simulink model "PID_Yaw_2018b"  (R2023a)
settings: Solver=ode3  StartTime=0.0  StopTime=inf  FixedStep=.02  RelTol=1e-3  EnableMultiTasking=on
InitFcn:
  | close all
  | clear
  | clc
  | Parameter_Modeling
  | ST=0.02;
  | angle_scale=.0109863;  % 1/91.0222
  | time_scale=.01;
values from neighbouring files (symbols this model uses):
  b = 1.10794e-05    [disturbance result.mat]
  d = reshape([p1dot;p2dot],2 * n^2,1)    [OpenLoop_LQDG_riccati_solver_pitch.m]    (also in OpenLoop_LQDG_riccati_solver_roll.m; disturbance result.mat = 3.2e-06)
undefined symbols (not defined in the file or in its folder): dcg, I_XX, I_YY, I_ZZ, rad, s
libraries: arduinolib x5, aerolibconvert2 x5
settings Model: SimulationMode=external  ExtModeTrigDuration=2  Creator=Alireza  LastModifiedBy=Ali
settings SolverCC: AlgebraicLoopSolver=TrustRegion
settings DataIOCC: LimitDataPoints=on  SaveFormat=Array  ReturnWorkspaceOutputs=off
settings OptimizationCC: ExpressionDepthLimit=2147483647  MaxStackSize=64  EfficientTunableParamExpr=on
settings DebuggingCC: UnderspecifiedInitializationDetection=Classic  MergeDetectMultiDrivingBlocksExec=none  ParameterTunabilityLossMsg=error  UnconnectedInputMsg=warning  UnconnectedOutputMsg=warning  UnconnectedLineMsg=warning  StateNameClashWarn=warning  SFUnexpectedBacktrackingDiag=warning  SFNoUnconditionalDefaultTransitionDiag=warning  SFExecutionAtInitializationDiag=none  ArithmeticOperatorsInVariantConditions=warning
settings HardwareCC: ProdBitPerInt=16  ProdBitPerPointer=16  ProdBitPerSizeT=16  ProdBitPerPtrDiffT=16  ProdLargestAtomicFloat=None  ProdWordSize=8  ProdHWDeviceType=Atmel->AVR
settings ModelReferenceCC: EnableRefExpFcnMdlSchedulingChecks=on  PropagateSignalLabelsOutOfModel=off
settings SFSimCC: SimUseLocalCustomCode=off  MATLABDynamicMemAlloc=off  CustomCodeUndefinedFunction=UseInterfaceOnly
settings RTWCC: Description=Embedded Coder  SystemTargetFile=ert.tlc  HardwareBoard=Arduino Mega 2560  TLCOptions=-aInlineSetEventsForThisBaseRateFcn=TLC_FALSE -aRateBasedStepFcn=1 -aSuppressMultiTaskScheduler=TLC_FALSE  TemplateMakefile=ert_default_tmf  GenerateReport=on  RTWVerbose=off  RTWUseLocalCustomCode=off  Toolchain=Arduino AVR  BuildConfiguration=Faster Runs  IncludeHyperlinkInReport=on  LaunchReport=on  GenerateTraceInfo=on  GenerateTraceReport=on  GenerateTraceReportSl=on  GenerateTraceReportSf=on  GenerateTraceReportEml=on
settings CodeAppCC: ForceParamTrailComments=on  IgnoreCustomStorageClasses=off  OperatorAnnotations=on  SimulinkDataObjDesc=on  SFDataObjDesc=on  MATLABFcnDesc=on  CustomSymbolStrType=$N$R$M  InsertBlockDesc=on  StateflowObjectComments=on  MATLABSourceComments=on  InternalIdentifier=Classic
settings ERTTargetCC: MultiwordLength=2048  SupportContinuousTime=on  SupportVariableSizeSignals=on
settings ConfigComp: CovMetricSettings=dw  CovSaveCumulativeToWorkspaceVar=on  CovSaveSingleToWorkspaceVar=on  CovExternalEMLEnable=off  CovSFcnEnable=off

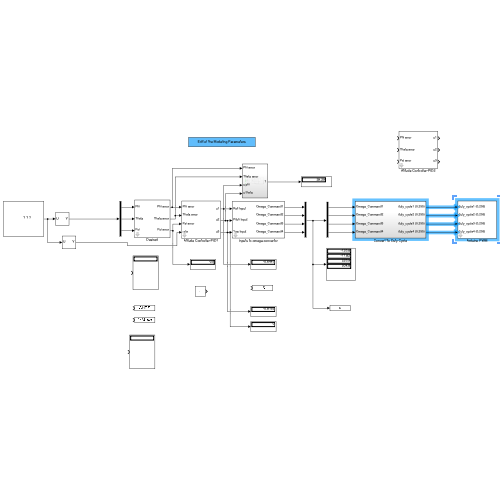
[thumbnail: Simulink's stored preview of the top-level diagram]
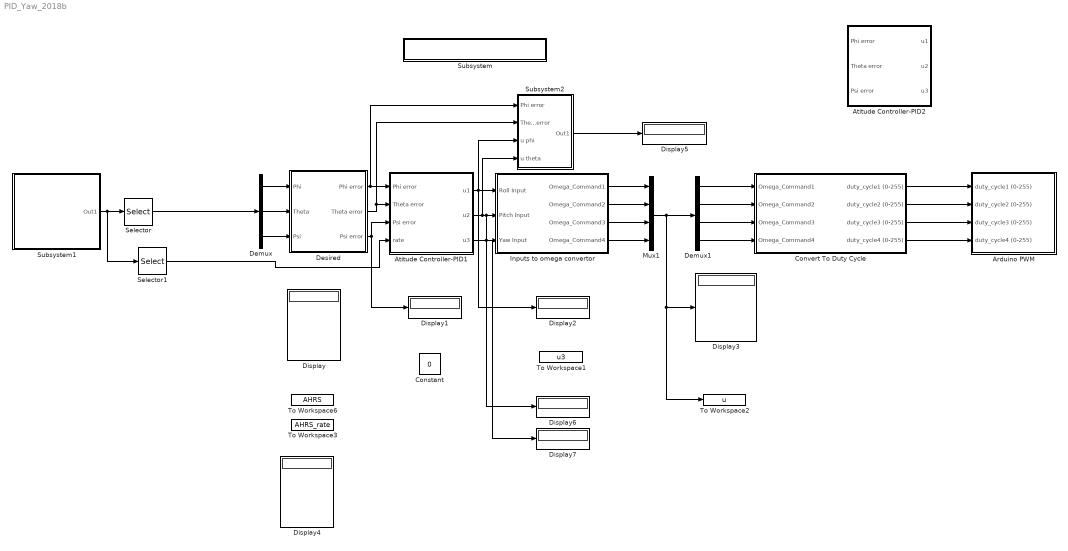
== system PID_Yaw_2018b ==
  Arduino PWM : Subsystem  mask{Motor1=8, Motor2=9, Motor3=10, Motor4=11}
      mask prompts: Motor1 "Motor 1 Pin Number"; Motor2 "Motor 2 Pin Number"; Motor3 "Motor 3 Pin Number"; Motor4 "Motor 4 Pin Number"
  Atitude Controller-PID1 : Subsystem  mask{KP_Roll=0.7, KI_Roll=0.5, KD_Roll=0.4, KP_Pitch=0.8, KI_Pitch=0.6, KD_Pitch=0.5, KP_Yaw=0, KI_Yaw=0, KD_Yaw=0}
      mask DialogControl tab1 Prompt: Roll
      mask DialogControl tab2 Prompt: Pitch
      mask DialogControl tab3 Prompt: Yaw
  Atitude Controller-PID2 : Subsystem  mask{KP_Roll=0.7, KI_Roll=0.5, KD_Roll=.4, KP_Pitch=.8, KI_Pitch=0.5, KD_Pitch=.4, KP_Yaw=0, KI_Yaw=0, KD_Yaw=0}
      mask DialogControl tab1 Prompt: Roll
      mask DialogControl tab2 Prompt: Pitch
      mask DialogControl tab3 Prompt: Yaw
  Constant : Constant  Value=0
  Convert To Duty Cycle : Subsystem
  Demux : Demux  Outputs=3
  Demux1 : Demux
  Desired : Subsystem  mask{Phi_Des=0, Theta_Des=0, Psi_Des=0}
      mask prompts: Phi_Des "Desired Phi (Degree)"; Theta_Des "Desired Theta (Degree)"; Psi_Des "Desired Psi (Degree)"
  Display{,1..7} (8 alike) : Display
  Inputs to omega convertor : Subsystem  mask{mean_rpm=2000}
  Mux1 : Mux
  Selector : Selector  InputPortWidth=6  IndexOptions=Index vector (dialog)  Indices=[1 2 3]  OutputSizes=1
  Selector1 : Selector  InputPortWidth=6  IndexOptions=Index vector (dialog)  Indices=[4 5 6]  OutputSizes=1
  Subsystem : Subsystem
      settings: OpenFcn=open('Parameter_Modeling')
      mask Display: disp('Edit of the Modeling Parameters')
  Subsystem1 : Subsystem
      mask Display: image('UM7.jpg'); % Use "Edit Image" on toolstrip to change.
  Subsystem2 : Subsystem
  To Workspace1 : ToWorkspace  VariableName=u3  SampleTime=-1
  To Workspace2 : ToWorkspace  VariableName=u  SampleTime=-1
  To Workspace3 : ToWorkspace  VariableName=AHRS_rate  SampleTime=-1
  To Workspace6 : ToWorkspace  VariableName=AHRS  SampleTime=-1
  wires:
  Desired/1(Phi error) -> Subsystem2/1(Phi error), Atitude Controller-PID1/1(Phi error)
  Desired/2(Theta error) -> Subsystem2/2(Theta error), Atitude Controller-PID1/2(Theta error)
  Desired/3(Psi error) -> Display1/1, Atitude Controller-PID1/3(Psi error)
  Convert To Duty Cycle/3(duty_cycle3 (0-255)) -> Arduino PWM/3(duty_cycle3 (0-255))
  Convert To Duty Cycle/1(duty_cycle1 (0-255)) -> Arduino PWM/1(duty_cycle1 (0-255))
  Convert To Duty Cycle/4(duty_cycle4 (0-255)) -> Arduino PWM/4(duty_cycle4 (0-255))
  Convert To Duty Cycle/2(duty_cycle2 (0-255)) -> Arduino PWM/2(duty_cycle2 (0-255))
  Demux/2 -> Desired/2(Theta)
  Demux/1 -> Desired/1(Phi)
  Demux/3 -> Desired/3(Psi)
  Mux1/1 -> Demux1/1, To Workspace2/1, Display3/1
  Inputs to omega convertor/2(Omega_Command2) -> Mux1/2
  Inputs to omega convertor/4(Omega_Command4) -> Mux1/4
  Inputs to omega convertor/3(Omega_Command3) -> Mux1/3
  Inputs to omega convertor/1(Omega_Command1) -> Mux1/1
  Demux1/4 -> Convert To Duty Cycle/4(Omega_Command4)
  Demux1/2 -> Convert To Duty Cycle/2(Omega_Command2)
  Demux1/3 -> Convert To Duty Cycle/3(Omega_Command3)
  Demux1/1 -> Convert To Duty Cycle/1(Omega_Command1)
  Subsystem1/1(Out1) -> Selector1/1, Selector/1
  Selector1/1 -> Atitude Controller-PID1/4(rate)
  Atitude Controller-PID1/1(u1) -> Display2/1, Subsystem2/3(u phi), Inputs to omega convertor/1(Roll Input)
  Atitude Controller-PID1/2(u2) -> Subsystem2/4(u theta), Display6/1, Inputs to omega convertor/2(Pitch Input)
  Atitude Controller-PID1/3(u3) -> Display7/1, Inputs to omega convertor/3(Yaw Input)
  Subsystem2/1(Out1) -> Display5/1
  Selector/1 -> Demux/1

== system PID_Yaw_2018b/Arduino PWM ==
  duty_cycle1 (0-255) : Inport
  duty_cycle2 (0-255) : Inport  Port=2
  duty_cycle3 (0-255) : Inport  Port=3
  duty_cycle4 (0-255) : Inport  Port=4
  PWM : arduinolib/PWM  pinNumber=8  frequencyType=Default  desiredFrequency=490.2  achievableFrequency=490.2
  PWM1 : arduinolib/PWM  pinNumber=9  frequencyType=Default  desiredFrequency=490.2  achievableFrequency=490.2
  PWM2 : arduinolib/PWM  pinNumber=10  frequencyType=Default  desiredFrequency=490.2  achievableFrequency=490.2
  PWM3 : arduinolib/PWM  pinNumber=11  frequencyType=Default  desiredFrequency=490.2  achievableFrequency=490.2
  wires:
  duty_cycle1 (0-255)/1 -> PWM/1
  duty_cycle2 (0-255)/1 -> PWM1/1
  duty_cycle3 (0-255)/1 -> PWM2/1
  duty_cycle4 (0-255)/1 -> PWM3/1

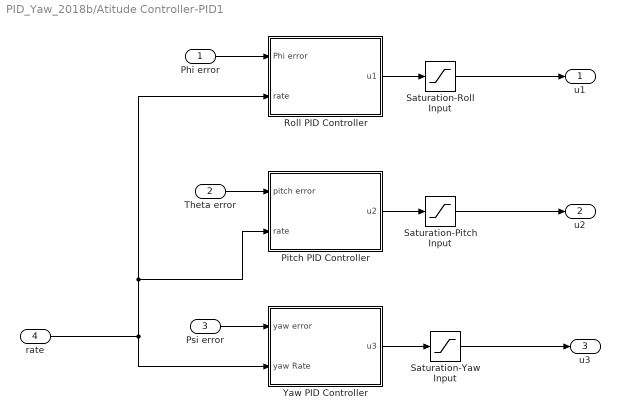
== system PID_Yaw_2018b/Atitude Controller-PID1 ==
  Phi error : Inport
  Theta error : Inport  Port=2
  Psi error : Inport  Port=3
  rate : Inport  Port=4
  Pitch PID Controller : Subsystem
  Roll PID Controller : Subsystem
  Saturation-Pitch Input : Saturate  UpperLimit=2  LowerLimit=-2
  Saturation-Roll Input : Saturate  UpperLimit=2  LowerLimit=-2
  Saturation-Yaw Input : Saturate  UpperLimit=2  LowerLimit=-2
  Yaw PID Controller : Subsystem
  u1 : Outport
  u2 : Outport  Port=2
  u3 : Outport  Port=3
  wires:
  Yaw PID Controller/1(u3) -> Saturation-Yaw Input/1
  Pitch PID Controller/1(u2) -> Saturation-Pitch Input/1
  Roll PID Controller/1(u1) -> Saturation-Roll Input/1
  Saturation-Roll Input/1 -> u1/1
  Psi error/1 -> Yaw PID Controller/1(yaw error)
  Theta error/1 -> Pitch PID Controller/1(pitch error)
  Phi error/1 -> Roll PID Controller/1(Phi error)
  rate/1 -> Pitch PID Controller/2(rate), Roll PID Controller/2(rate), Yaw PID Controller/2(yaw Rate)
  Saturation-Pitch Input/1 -> u2/1
  Saturation-Yaw Input/1 -> u3/1

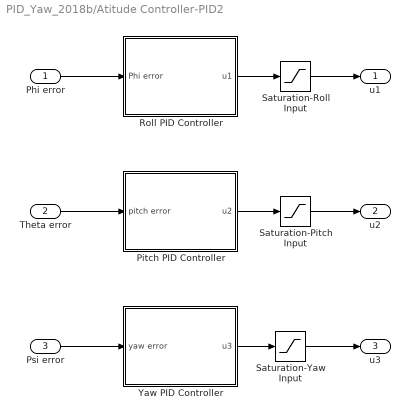
== system PID_Yaw_2018b/Atitude Controller-PID2 ==
  Phi error : Inport
  Theta error : Inport  Port=2
  Psi error : Inport  Port=3
  Pitch PID Controller : Subsystem
  Roll PID Controller : Subsystem
  Saturation-Pitch Input : Saturate  UpperLimit=2  LowerLimit=-2
  Saturation-Roll Input : Saturate  UpperLimit=2  LowerLimit=-2
  Saturation-Yaw Input : Saturate  UpperLimit=2  LowerLimit=-2
  Yaw PID Controller : Subsystem
  u1 : Outport
  u2 : Outport  Port=2
  u3 : Outport  Port=3
  wires:
  Yaw PID Controller/1(u3) -> Saturation-Yaw Input/1
  Pitch PID Controller/1(u2) -> Saturation-Pitch Input/1
  Roll PID Controller/1(u1) -> Saturation-Roll Input/1
  Saturation-Yaw Input/1 -> u3/1
  Saturation-Roll Input/1 -> u1/1
  Saturation-Pitch Input/1 -> u2/1
  Psi error/1 -> Yaw PID Controller/1(yaw error)
  Theta error/1 -> Pitch PID Controller/1(pitch error)
  Phi error/1 -> Roll PID Controller/1(Phi error)

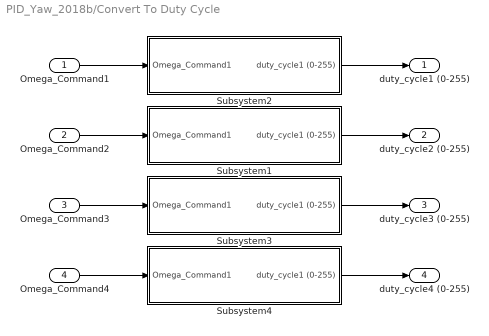
== system PID_Yaw_2018b/Convert To Duty Cycle ==
  Omega_Command1 : Inport
  Omega_Command2 : Inport  Port=2
  Omega_Command3 : Inport  Port=3
  Omega_Command4 : Inport  Port=4
  Subsystem1 : Subsystem
  Subsystem2 : Subsystem
  Subsystem3 : Subsystem
  Subsystem4 : Subsystem
  duty_cycle1 (0-255) : Outport
  duty_cycle2 (0-255) : Outport  Port=2
  duty_cycle3 (0-255) : Outport  Port=3
  duty_cycle4 (0-255) : Outport  Port=4
  wires:
  Subsystem1/1(duty_cycle1 (0-255)) -> duty_cycle2 (0-255)/1
  Subsystem3/1(duty_cycle1 (0-255)) -> duty_cycle3 (0-255)/1
  Subsystem4/1(duty_cycle1 (0-255)) -> duty_cycle4 (0-255)/1
  Subsystem2/1(duty_cycle1 (0-255)) -> duty_cycle1 (0-255)/1
  Omega_Command1/1 -> Subsystem2/1(Omega_Command1)
  Omega_Command4/1 -> Subsystem4/1(Omega_Command1)
  Omega_Command3/1 -> Subsystem3/1(Omega_Command1)
  Omega_Command2/1 -> Subsystem1/1(Omega_Command1)

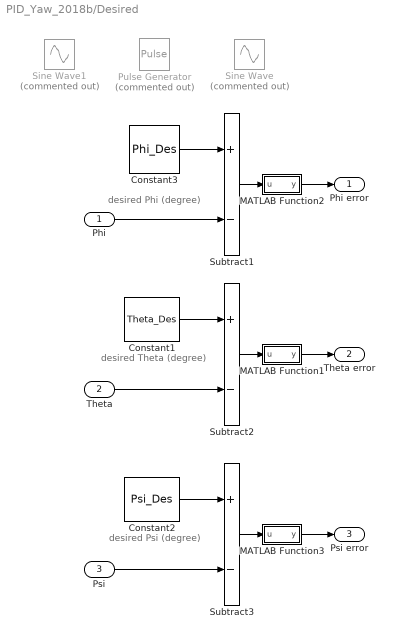
== system PID_Yaw_2018b/Desired ==
  note: desired Phi (degree)
  note: desired Theta (degree)
  note: desired Psi (degree)
  Phi : Inport
  Theta : Inport  Port=2
  Psi : Inport  Port=3
  Constant1 : Constant  Value=Theta_Des
  Constant2 : Constant  Value=Psi_Des
  Constant3 : Constant  Value=Phi_Des
  MATLAB Function1 : MATLAB Function  TreatAsAtomicUnit=on
  MATLAB Function2 : MATLAB Function  TreatAsAtomicUnit=on
  MATLAB Function3 : MATLAB Function  TreatAsAtomicUnit=on
  Pulse Generator : DiscretePulseGenerator  Commented=on  PulseType=Time based  Amplitude=20  Period=10  PulseWidth=5
  Sine Wave : Sin  Commented=on  Amplitude=10  SampleTime=0
  Sine Wave1 : Sin  Commented=on  Amplitude=20  Phase=pi/2  SampleTime=0
  Subtract1 : Sum  Inputs=+-
  Subtract2 : Sum  Inputs=+-
  Subtract3 : Sum  Inputs=+-
  Phi error : Outport
  Theta error : Outport  Port=2
  Psi error : Outport  Port=3
  wires:
  Constant2/1 -> Subtract3/1
  Psi/1 -> Subtract3/2
  Subtract2/1 -> MATLAB Function1/1(u)
  Theta/1 -> Subtract2/2
  Subtract1/1 -> MATLAB Function2/1(u)
  Phi/1 -> Subtract1/2
  Subtract3/1 -> MATLAB Function3/1(u)
  MATLAB Function2/1(y) -> Phi error/1
  MATLAB Function1/1(y) -> Theta error/1
  MATLAB Function3/1(y) -> Psi error/1
  Constant1/1 -> Subtract2/1
  Constant3/1 -> Subtract1/1

== system PID_Yaw_2018b/Inputs to omega convertor ==
  Roll Input : Inport
  Pitch Input : Inport  Port=2
  Yaw Input : Inport  Port=3
  " 1" : Constant  Value=mean_rpm
  Inputs to omega convertor : Subsystem
  Omega_Command1 : Outport
  Omega_Command2 : Outport  Port=2
  Omega_Command3 : Outport  Port=3
  Omega_Command4 : Outport  Port=4
  wires:
  " 1"/1 -> Inputs to omega convertor/1(mean rpm)
  Roll Input/1 -> Inputs to omega convertor/2(Roll Input (Roll Moment))
  Pitch Input/1 -> Inputs to omega convertor/3(Pitch Input (Pitch Moment))
  Yaw Input/1 -> Inputs to omega convertor/4(Yaw Input(Yaw Moment))
  Inputs to omega convertor/4(Omega_Command4) -> Omega_Command4/1
  Inputs to omega convertor/1(Omega_Command1) -> Omega_Command1/1
  Inputs to omega convertor/2(Omega_Command2) -> Omega_Command2/1
  Inputs to omega convertor/3(Omega_Command3) -> Omega_Command3/1

== system PID_Yaw_2018b/Subsystem ==

== system PID_Yaw_2018b/Subsystem1 ==
  AHRS : Subsystem
  Mux : Mux  Inputs=6
  Out1 : Outport
  wires:
  AHRS/2(theta) -> Mux/2
  AHRS/1(phi) -> Mux/1
  AHRS/3(psi) -> Mux/3
  AHRS/4(roll_rate) -> Mux/4
  AHRS/5(pitch_rate) -> Mux/5
  AHRS/6(yaw_rate) -> Mux/6
  Mux/1 -> Out1/1

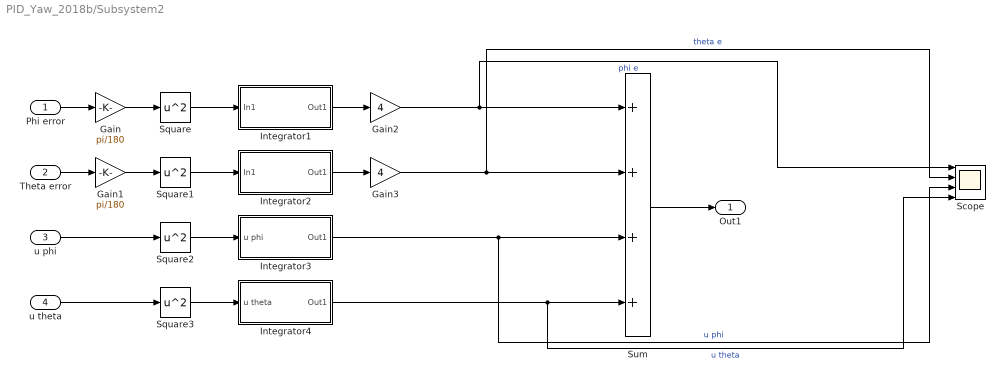
== system PID_Yaw_2018b/Subsystem2 ==
  Phi error : Inport
  Theta error : Inport  Port=2
  u phi : Inport  Port=3
  u theta : Inport  Port=4
  Gain : Gain  Gain=pi/180
  Gain1 : Gain  Gain=pi/180
  Gain2 : Gain  Gain=4
  Gain3 : Gain  Gain=4
  Integrator1 : Subsystem
  Integrator2 : Subsystem
  Integrator3 : Subsystem
  Integrator4 : Subsystem
  Scope : Scope  NumInputPorts=4
  Square{,1..3} (4 alike) : Math  Operator=square
  Sum : Sum  Inputs=++++
  Out1 : Outport
  wires:
  Sum/1 -> Out1/1
  Integrator1/1(Out1) -> Gain2/1
  Integrator2/1(Out1) -> Gain3/1
  Integrator3/1(Out1) -> Scope/3, Sum/3  "u phi"
  Integrator4/1(Out1) -> Scope/4, Sum/4  "u theta"
  Gain/1 -> Square/1
  Phi error/1 -> Gain/1
  Theta error/1 -> Gain1/1
  Gain1/1 -> Square1/1
  u phi/1 -> Square2/1
  u theta/1 -> Square3/1
  Square/1 -> Integrator1/1(In1)
  Square1/1 -> Integrator2/1(In1)
  Square2/1 -> Integrator3/1(u phi)
  Square3/1 -> Integrator4/1(u theta)
  Gain2/1 -> Scope/1, Sum/1  "phi e"
  Gain3/1 -> Scope/2, Sum/2  "theta e"

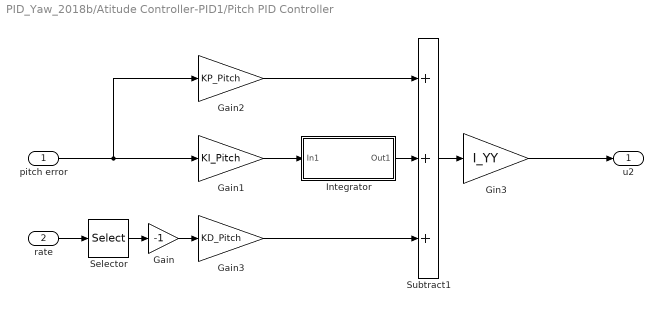
== system PID_Yaw_2018b/Atitude Controller-PID1/Pitch PID Controller ==
  pitch error : Inport
  rate : Inport  Port=2
  Gain : Gain  Gain=-1
  Gain1 : Gain  Gain=KI_Pitch
  Gain2 : Gain  Gain=KP_Pitch
  Gain3 : Gain  Gain=KD_Pitch
  Gin3 : Gain  Gain=I_YY
  Integrator : Subsystem
  Selector : Selector  InputPortWidth=3  IndexOptions=Index vector (dialog)  Indices=[2]  OutputSizes=1
  Subtract1 : Sum  Inputs=+++
  u2 : Outport
  wires:
  Integrator/1(Out1) -> Subtract1/2
  Gain1/1 -> Integrator/1(In1)
  Gain2/1 -> Subtract1/1
  Subtract1/1 -> Gin3/1
  Gain/1 -> Gain3/1
  pitch error/1 -> Gain1/1, Gain2/1
  Gin3/1 -> u2/1
  Gain3/1 -> Subtract1/3
  rate/1 -> Selector/1
  Selector/1 -> Gain/1

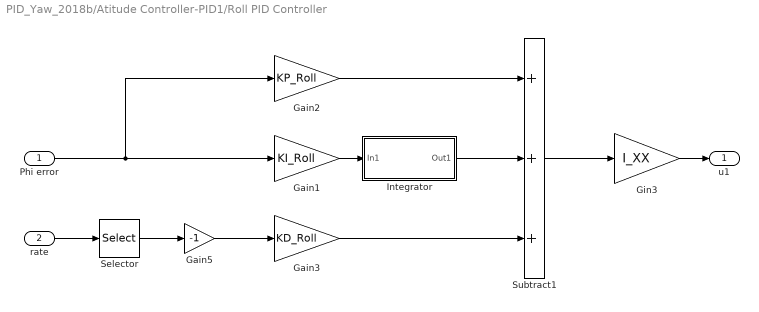
== system PID_Yaw_2018b/Atitude Controller-PID1/Roll PID Controller ==
  Phi error : Inport
  rate : Inport  Port=2
  Gain1 : Gain  Gain=KI_Roll
  Gain2 : Gain  Gain=KP_Roll
  Gain3 : Gain  Gain=KD_Roll
  Gain5 : Gain  Gain=-1
  Gin3 : Gain  Gain=I_XX
  Integrator : Subsystem
  Selector : Selector  InputPortWidth=3  IndexOptions=Index vector (dialog)  Indices=[1]  OutputSizes=1
  Subtract1 : Sum  Inputs=+++
  u1 : Outport
  wires:
  Gain1/1 -> Integrator/1(In1)
  Gin3/1 -> u1/1
  Gain2/1 -> Subtract1/1
  Subtract1/1 -> Gin3/1
  Integrator/1(Out1) -> Subtract1/2
  rate/1 -> Selector/1
  Phi error/1 -> Gain1/1, Gain2/1
  Selector/1 -> Gain5/1
  Gain3/1 -> Subtract1/3
  Gain5/1 -> Gain3/1

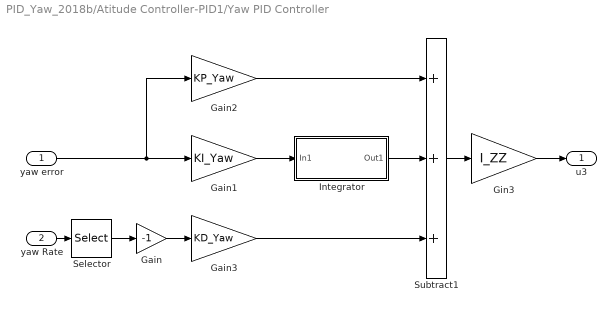
== system PID_Yaw_2018b/Atitude Controller-PID1/Yaw PID Controller ==
  yaw error : Inport
  yaw Rate : Inport  Port=2
  Gain : Gain  Gain=-1
  Gain1 : Gain  Gain=KI_Yaw
  Gain2 : Gain  Gain=KP_Yaw
  Gain3 : Gain  Gain=KD_Yaw
  Gin3 : Gain  Gain=I_ZZ
  Integrator : Subsystem
  Selector : Selector  InputPortWidth=3  IndexOptions=Index vector (dialog)  Indices=[3]  OutputSizes=1
  Subtract1 : Sum  Inputs=+++
  u3 : Outport
  wires:
  Gain3/1 -> Subtract1/3
  Integrator/1(Out1) -> Subtract1/2
  Gain1/1 -> Integrator/1(In1)
  Gin3/1 -> u3/1
  Gain2/1 -> Subtract1/1
  yaw error/1 -> Gain2/1, Gain1/1
  Subtract1/1 -> Gin3/1
  yaw Rate/1 -> Selector/1
  Selector/1 -> Gain/1
  Gain/1 -> Gain3/1

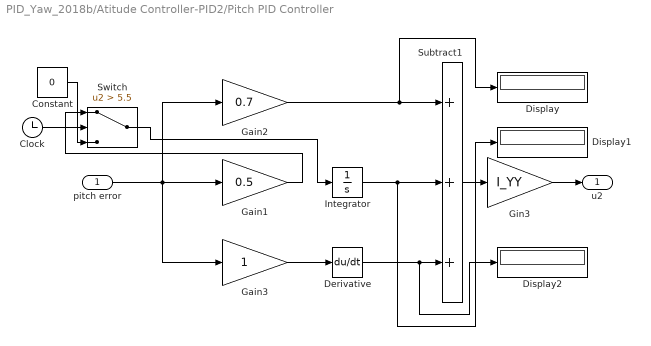
== system PID_Yaw_2018b/Atitude Controller-PID2/Pitch PID Controller ==
  pitch error : Inport
  Clock : Clock
  Constant : Constant  Value=0
  Derivative : Derivative
  Display : Display
  Display1 : Display
  Display2 : Display
  Gain1 : Gain  Gain=0.5
  Gain2 : Gain  Gain=0.7
  Gain3 : Gain
  Gin3 : Gain  Gain=I_YY
  Integrator : Integrator  LimitOutput=on  UpperSaturationLimit=10  LowerSaturationLimit=-10
  Subtract1 : Sum  Inputs=+++
  Switch : Switch  Criteria=u2 > Threshold  Threshold=5.5  SaturateOnIntegerOverflow=off  InputSameDT=off
  u2 : Outport
  wires:
  Gain3/1 -> Derivative/1
  Integrator/1 -> Display1/1, Subtract1/2
  Derivative/1 -> Display2/1, Subtract1/3
  Gin3/1 -> u2/1
  Gain2/1 -> Display/1, Subtract1/1
  pitch error/1 -> Gain2/1, Gain1/1, Gain3/1
  Subtract1/1 -> Gin3/1
  Clock/1 -> Switch/2
  Switch/1 -> Integrator/1
  Gain1/1 -> Switch/1
  Constant/1 -> Switch/3

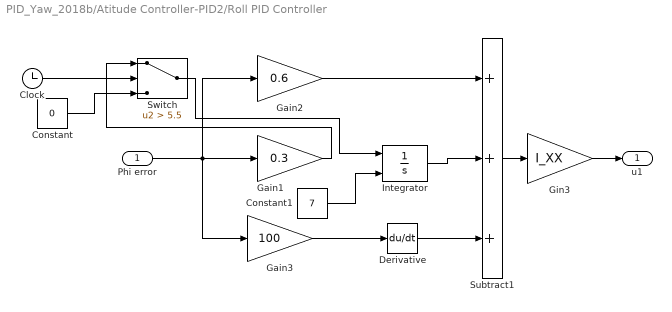
== system PID_Yaw_2018b/Atitude Controller-PID2/Roll PID Controller ==
  Phi error : Inport
  Clock : Clock
  Constant : Constant  Value=0
  Constant1 : Constant  Value=7
  Derivative : Derivative
  Gain1 : Gain  Gain=0.3
  Gain2 : Gain  Gain=0.6
  Gain3 : Gain  Gain=100
  Gin3 : Gain  Gain=I_XX
  Integrator : Integrator  ExternalReset=rising  LimitOutput=on  UpperSaturationLimit=10  LowerSaturationLimit=-10
  Subtract1 : Sum  Inputs=+++
  Switch : Switch  Criteria=u2 > Threshold  Threshold=5.5  SaturateOnIntegerOverflow=off  InputSameDT=off
  u1 : Outport
  wires:
  Integrator/1 -> Subtract1/2
  Gain3/1 -> Derivative/1
  Gin3/1 -> u1/1
  Phi error/1 -> Gain2/1, Gain3/1, Gain1/1
  Gain2/1 -> Subtract1/1
  Subtract1/1 -> Gin3/1
  Derivative/1 -> Subtract1/3
  Clock/1 -> Switch/2
  Gain1/1 -> Switch/1
  Switch/1 -> Integrator/1
  Constant/1 -> Switch/3
  Constant1/1 -> Integrator/2

== system PID_Yaw_2018b/Atitude Controller-PID2/Yaw PID Controller ==
  yaw error : Inport
  Derivative : Derivative
  Gain1 : Gain  Gain=KI_Yaw
  Gain2 : Gain  Gain=KP_Yaw
  Gain3 : Gain  Gain=KD_Yaw
  Gin3 : Gain  Gain=I_ZZ
  Integrator : Integrator  LimitOutput=on  UpperSaturationLimit=10  LowerSaturationLimit=-10
  Subtract1 : Sum  Inputs=+++
  u3 : Outport
  wires:
  Derivative/1 -> Subtract1/3
  Integrator/1 -> Subtract1/2
  Gain1/1 -> Integrator/1
  Gain3/1 -> Derivative/1
  Gin3/1 -> u3/1
  Gain2/1 -> Subtract1/1
  yaw error/1 -> Gain2/1, Gain1/1, Gain3/1
  Subtract1/1 -> Gin3/1

== system PID_Yaw_2018b/Convert To Duty Cycle/Subsystem1 ==
  Omega_Command1 : Inport
  Angular Velocity Conversion : aerolibconvert2/Angular Velocity Conversion  IU=rad/s  OU=rpm
  Clock : Clock
  Constant4 : Constant  Value=255
  Divide1 : Product  Inputs=**
  Saturation : Saturate  UpperLimit=6000  LowerLimit=1300
  Starter : Subsystem
  Switch : Switch  Criteria=u2 > Threshold  Threshold=5  SaturateOnIntegerOverflow=off  InputSameDT=off
  rpm2duty_Emax : Lookup_n-D  NumberOfTableDimensions=1  BreakpointsForDimension1=|  Table=|  RndMeth=Simplest
      BreakpointsForDimension1=|
      | [1201
      | 2305
      | 3096
      | 3930
      | 4118
      | 4555
      | 5122
      | 5552
      | 5957
      | 6291
      | 6360]
      Table=|
      | [0.5
      | 0.55
      | 0.6
      | 0.65
      | 0.7
      | 0.75
      | 0.8
      | 0.85
      | 0.9
      | 0.95
      | 1]
  duty_cycle1 (0-255) : Outport
  wires:
  Divide1/1 -> Switch/1
  Switch/1 -> duty_cycle1 (0-255)/1
  Clock/1 -> Switch/2
  Starter/1(start_pulse) -> Switch/3
  Angular Velocity Conversion/1 -> Saturation/1
  Constant4/1 -> Divide1/2
  Omega_Command1/1 -> Angular Velocity Conversion/1
  rpm2duty_Emax/1 -> Divide1/1
  Saturation/1 -> rpm2duty_Emax/1

== system PID_Yaw_2018b/Convert To Duty Cycle/Subsystem2 ==
  Omega_Command1 : Inport
  Angular Velocity Conversion : aerolibconvert2/Angular Velocity Conversion  IU=rad/s  OU=rpm
  Clock : Clock
  Constant4 : Constant  Value=255
  Divide1 : Product  Inputs=**
  Saturation : Saturate  UpperLimit=6000  LowerLimit=1300
  Starter : Subsystem
  Switch : Switch  Criteria=u2 > Threshold  Threshold=5  SaturateOnIntegerOverflow=off  InputSameDT=off
  rpm2duty_Emax : Lookup_n-D  NumberOfTableDimensions=1  BreakpointsForDimension1=|  Table=|  RndMeth=Simplest
      BreakpointsForDimension1=|
      | [1201
      | 2305
      | 3096
      | 3930
      | 4118
      | 4555
      | 5122
      | 5552
      | 5957
      | 6291
      | 6360]
      Table=|
      | [0.5
      | 0.55
      | 0.6
      | 0.65
      | 0.7
      | 0.75
      | 0.8
      | 0.85
      | 0.9
      | 0.95
      | 1]
  duty_cycle1 (0-255) : Outport
  wires:
  Omega_Command1/1 -> Angular Velocity Conversion/1
  Constant4/1 -> Divide1/2
  Angular Velocity Conversion/1 -> Saturation/1
  Starter/1(start_pulse) -> Switch/3
  Clock/1 -> Switch/2
  Switch/1 -> duty_cycle1 (0-255)/1
  Divide1/1 -> Switch/1
  rpm2duty_Emax/1 -> Divide1/1
  Saturation/1 -> rpm2duty_Emax/1

== system PID_Yaw_2018b/Convert To Duty Cycle/Subsystem3 ==
  Omega_Command1 : Inport
  Angular Velocity Conversion : aerolibconvert2/Angular Velocity Conversion  IU=rad/s  OU=rpm
  Clock : Clock
  Constant4 : Constant  Value=255
  Divide1 : Product  Inputs=**
  Saturation : Saturate  UpperLimit=6000  LowerLimit=1300
  Starter : Subsystem
  Switch : Switch  Criteria=u2 > Threshold  Threshold=5  SaturateOnIntegerOverflow=off  InputSameDT=off
  rpm2duty_Emax : Lookup_n-D  NumberOfTableDimensions=1  BreakpointsForDimension1=|  Table=|  RndMeth=Simplest
      BreakpointsForDimension1=|
      | [1201
      | 2305
      | 3096
      | 3930
      | 4118
      | 4555
      | 5122
      | 5552
      | 5957
      | 6291
      | 6360]
      Table=|
      | [0.5
      | 0.55
      | 0.6
      | 0.65
      | 0.7
      | 0.75
      | 0.8
      | 0.85
      | 0.9
      | 0.95
      | 1]
  duty_cycle1 (0-255) : Outport
  wires:
  Omega_Command1/1 -> Angular Velocity Conversion/1
  Constant4/1 -> Divide1/2
  Angular Velocity Conversion/1 -> Saturation/1
  Starter/1(start_pulse) -> Switch/3
  Clock/1 -> Switch/2
  Switch/1 -> duty_cycle1 (0-255)/1
  Divide1/1 -> Switch/1
  rpm2duty_Emax/1 -> Divide1/1
  Saturation/1 -> rpm2duty_Emax/1

== system PID_Yaw_2018b/Convert To Duty Cycle/Subsystem4 ==
  Omega_Command1 : Inport
  Angular Velocity Conversion : aerolibconvert2/Angular Velocity Conversion  IU=rad/s  OU=rpm
  Clock : Clock
  Constant4 : Constant  Value=255
  Divide1 : Product  Inputs=**
  Saturation : Saturate  UpperLimit=6000  LowerLimit=1300
  Starter : Subsystem
  Switch : Switch  Criteria=u2 > Threshold  Threshold=5  SaturateOnIntegerOverflow=off  InputSameDT=off
  rpm2duty_Emax : Lookup_n-D  NumberOfTableDimensions=1  BreakpointsForDimension1=|  Table=|  RndMeth=Simplest
      BreakpointsForDimension1=|
      | [1201
      | 2305
      | 3096
      | 3930
      | 4118
      | 4555
      | 5122
      | 5552
      | 5957
      | 6291
      | 6360]
      Table=|
      | [0.5
      | 0.55
      | 0.6
      | 0.65
      | 0.7
      | 0.75
      | 0.8
      | 0.85
      | 0.9
      | 0.95
      | 1]
  duty_cycle1 (0-255) : Outport
  wires:
  Divide1/1 -> Switch/1
  Switch/1 -> duty_cycle1 (0-255)/1
  Clock/1 -> Switch/2
  Starter/1(start_pulse) -> Switch/3
  Angular Velocity Conversion/1 -> Saturation/1
  Constant4/1 -> Divide1/2
  Omega_Command1/1 -> Angular Velocity Conversion/1
  rpm2duty_Emax/1 -> Divide1/1
  Saturation/1 -> rpm2duty_Emax/1

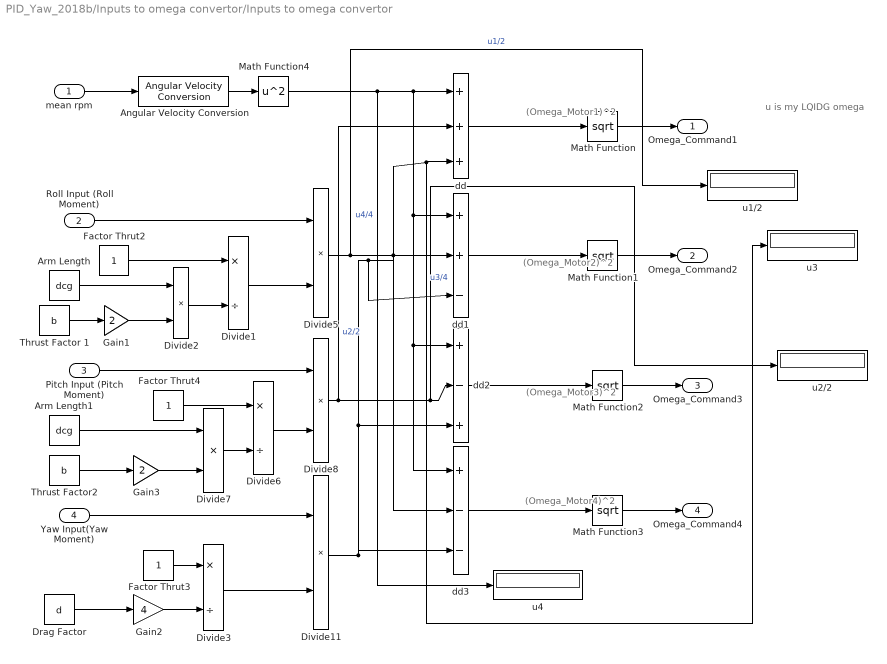
== system PID_Yaw_2018b/Inputs to omega convertor/Inputs to omega convertor ==
  note: u is my LQIDG omega
  note: (Omega_Motor4)^2
  note: (Omega_Motor3)^2
  note: (Omega_Motor2)^2
  note: (Omega_Motor1)^2
  mean rpm : Inport
  Roll Input (Roll Moment) : Inport  Port=2
  Pitch Input (Pitch Moment) : Inport  Port=3
  Yaw Input(Yaw Moment) : Inport  Port=4
  " Thrust Factor2" : Constant  Value=b
  Angular Velocity Conversion : aerolibconvert2/Angular Velocity Conversion  IU=rpm  OU=rad/s
  Arm Length : Constant  Value=dcg
  Arm Length1 : Constant  Value=dcg
  Divide1 : Product  Inputs=*/
  Divide{2,5,7..8,11} (5 alike) : Product  Inputs=**
  Divide3 : Product  Inputs=*/
  Divide6 : Product  Inputs=*/
  "Drag Factor " : Constant  Value=d
  Factor Thrut2 : Constant
  Factor Thrut3 : Constant
  Factor Thrut4 : Constant
  Gain1 : Gain  Gain=2
  Gain2 : Gain  Gain=4
  Gain3 : Gain  Gain=2
  Math Function{,1..3} (4 alike) : Math  Operator=sqrt  SignedPower=on
  Math Function4 : Math  Operator=square  SignedPower=on
  Thrust Factor 1 : Constant  Value=b
  dd : Sum  Inputs=+++
  dd1 : Sum  Inputs=++-
  dd2 : Sum  Inputs=+-+
  dd3 : Sum  Inputs=+--
  u1/2 : Display
  u2/2 : Display
  u3 : Display
  u4 : Display
  Omega_Command1 : Outport
  Omega_Command2 : Outport  Port=2
  Omega_Command3 : Outport  Port=3
  Omega_Command4 : Outport  Port=4
  wires:
  dd1/1 -> Math Function1/1
  dd2/1 -> Math Function2/1
  dd3/1 -> Math Function3/1
  dd/1 -> Math Function/1
  Divide5/1 -> u1/2/1, dd1/2, dd3/2  "u1/2"
  Divide11/1 -> dd3/3, u3/1, dd/3, dd1/3, dd2/3  "u3/4"
  Math Function4/1 -> u4/1, dd/1, dd1/1, dd2/1, dd3/1  "u4/4"
  Divide3/1 -> Divide11/2
  Yaw Input(Yaw Moment)/1 -> Divide11/1
  Divide6/1 -> Divide8/2
  Pitch Input (Pitch Moment)/1 -> Divide8/1
  Arm Length1/1 -> Divide7/1
  Gain3/1 -> Divide7/2
  " Thrust Factor2"/1 -> Gain3/1
  Divide7/1 -> Divide6/2
  Factor Thrut4/1 -> Divide6/1
  Divide1/1 -> Divide5/2
  Roll Input (Roll Moment)/1 -> Divide5/1
  Gain2/1 -> Divide3/2
  "Drag Factor "/1 -> Gain2/1
  Factor Thrut3/1 -> Divide3/1
  Arm Length/1 -> Divide2/1
  Gain1/1 -> Divide2/2
  Thrust Factor 1/1 -> Gain1/1
  Divide2/1 -> Divide1/2
  Factor Thrut2/1 -> Divide1/1
  Math Function/1 -> Omega_Command1/1
  Math Function1/1 -> Omega_Command2/1
  Math Function2/1 -> Omega_Command3/1
  Math Function3/1 -> Omega_Command4/1
  Divide8/1 -> dd/2, u2/2/1, dd2/2  "u2/2"
  Angular Velocity Conversion/1 -> Math Function4/1
  mean rpm/1 -> Angular Velocity Conversion/1

== system PID_Yaw_2018b/Subsystem1/AHRS ==
  Cast To Double : DataTypeConversion  OutDataTypeStr=double  SaturateOnIntegerOverflow=off  RndMeth=Floor
  Display : Display
  Reshape : Reshape
  Serial Receive : arduinolib/Serial Receive  isARMArch=off  portNumber=1  DataType=uint8  Datalength=32  SampleTime=0.02  showOutStatus=on  blockPlatform=arduino
  data_parsing : MATLAB Function  TreatAsAtomicUnit=on
  phi : Outport
  theta : Outport  Port=2
  psi : Outport  Port=3
  roll_rate : Outport  Port=4
  pitch_rate : Outport  Port=5
  yaw_rate : Outport  Port=6
  wires:
  data_parsing/2(theta) -> theta/1
  data_parsing/3(psi) -> psi/1
  data_parsing/4(roll_rate) -> roll_rate/1
  Reshape/1 -> data_parsing/1(data_uint8)
  data_parsing/1(phi) -> phi/1
  data_parsing/5(pitch_rate) -> pitch_rate/1
  Serial Receive/2 -> Display/1, data_parsing/2(status)
  data_parsing/6(yaw_rate) -> yaw_rate/1
  Cast To Double/1 -> Reshape/1
  Serial Receive/1 -> Cast To Double/1

== system PID_Yaw_2018b/Subsystem2/Integrator1 ==
  In1 : Inport
  Clock : Clock
  Constant : Constant  Value=0
  Integrator1 : Integrator
  Switch : Switch  Criteria=u2 > Threshold  Threshold=5  SaturateOnIntegerOverflow=off  InputSameDT=off
  Out1 : Outport
  wires:
  Switch/1 -> Integrator1/1
  Constant/1 -> Switch/3
  In1/1 -> Switch/1
  Clock/1 -> Switch/2
  Integrator1/1 -> Out1/1

== system PID_Yaw_2018b/Subsystem2/Integrator2 ==
  In1 : Inport
  Clock : Clock
  Constant : Constant  Value=0
  Integrator1 : Integrator
  Switch : Switch  Criteria=u2 > Threshold  Threshold=5  SaturateOnIntegerOverflow=off  InputSameDT=off
  Out1 : Outport
  wires:
  Switch/1 -> Integrator1/1
  Constant/1 -> Switch/3
  In1/1 -> Switch/1
  Clock/1 -> Switch/2
  Integrator1/1 -> Out1/1

== system PID_Yaw_2018b/Subsystem2/Integrator3 ==
  u phi : Inport
  Clock : Clock
  Constant : Constant  Value=0
  Integrator1 : Integrator
  Switch : Switch  Criteria=u2 > Threshold  Threshold=5  SaturateOnIntegerOverflow=off  InputSameDT=off
  Out1 : Outport
  wires:
  Switch/1 -> Integrator1/1
  Constant/1 -> Switch/3
  u phi/1 -> Switch/1
  Clock/1 -> Switch/2
  Integrator1/1 -> Out1/1

== system PID_Yaw_2018b/Subsystem2/Integrator4 ==
  u theta : Inport
  Clock : Clock
  Constant : Constant  Value=0
  Integrator1 : Integrator
  Switch : Switch  Criteria=u2 > Threshold  Threshold=5  SaturateOnIntegerOverflow=off  InputSameDT=off
  Out1 : Outport
  wires:
  Switch/1 -> Integrator1/1
  Constant/1 -> Switch/3
  u theta/1 -> Switch/1
  Clock/1 -> Switch/2
  Integrator1/1 -> Out1/1

== system PID_Yaw_2018b/Atitude Controller-PID1/Pitch PID Controller/Integrator ==
  In1 : Inport
  Clock : Clock
  Constant : Constant  Value=0
  Display : Display
  Display1 : Display
  Integrator1 : Integrator  LimitOutput=on  UpperSaturationLimit=10  LowerSaturationLimit=-10
  Switch : Switch  Criteria=u2 > Threshold  Threshold=5  SaturateOnIntegerOverflow=off  InputSameDT=off
  Out1 : Outport
  wires:
  Integrator1/1 -> Display/1, Out1/1
  Clock/1 -> Switch/2
  In1/1 -> Switch/1
  Constant/1 -> Switch/3
  Switch/1 -> Integrator1/1

== system PID_Yaw_2018b/Atitude Controller-PID1/Roll PID Controller/Integrator ==
  In1 : Inport
  Clock : Clock
  Constant : Constant  Value=0
  Integrator1 : Integrator  LimitOutput=on  UpperSaturationLimit=10  LowerSaturationLimit=-10
  Switch : Switch  Criteria=u2 > Threshold  Threshold=5  SaturateOnIntegerOverflow=off  InputSameDT=off
  Out1 : Outport
  wires:
  Integrator1/1 -> Out1/1
  Clock/1 -> Switch/2
  In1/1 -> Switch/1
  Constant/1 -> Switch/3
  Switch/1 -> Integrator1/1

== system PID_Yaw_2018b/Atitude Controller-PID1/Yaw PID Controller/Integrator ==
  In1 : Inport
  Clock : Clock
  Constant : Constant  Value=0
  Display : Display
  Display1 : Display
  Integrator1 : Integrator  LimitOutput=on  UpperSaturationLimit=10  LowerSaturationLimit=-10
  Switch : Switch  Criteria=u2 > Threshold  Threshold=5  SaturateOnIntegerOverflow=off  InputSameDT=off
  Out1 : Outport
  wires:
  Integrator1/1 -> Display/1, Out1/1
  Clock/1 -> Switch/2
  In1/1 -> Switch/1
  Constant/1 -> Switch/3
  Switch/1 -> Integrator1/1

== system PID_Yaw_2018b/Convert To Duty Cycle/Subsystem1/Starter ==
  Add : Sum
  Step : Step  After=140
  Step1 : Step  Time=2  After=-30
  start_pulse : Outport
  wires:
  Add/1 -> start_pulse/1
  Step/1 -> Add/1
  Step1/1 -> Add/2

== system PID_Yaw_2018b/Convert To Duty Cycle/Subsystem2/Starter ==
  Add : Sum
  Step : Step  After=140
  Step1 : Step  Time=2  After=-30
  start_pulse : Outport
  wires:
  Add/1 -> start_pulse/1
  Step/1 -> Add/1
  Step1/1 -> Add/2

== system PID_Yaw_2018b/Convert To Duty Cycle/Subsystem3/Starter ==
  Add : Sum
  Step : Step  After=140
  Step1 : Step  Time=2  After=-30
  start_pulse : Outport
  wires:
  Add/1 -> start_pulse/1
  Step/1 -> Add/1
  Step1/1 -> Add/2

== system PID_Yaw_2018b/Convert To Duty Cycle/Subsystem4/Starter ==
  Add : Sum
  Step : Step  After=140
  Step1 : Step  Time=2  After=-30
  start_pulse : Outport
  wires:
  Add/1 -> start_pulse/1
  Step/1 -> Add/1
  Step1/1 -> Add/2

== matlab function PID_Yaw_2018b/Subsystem1/AHRS/data_parsing ==
  data: phi output size=1; data_uint8 input size=32; theta output size=1; psi output size=1; roll_rate output size=1; pitch_rate output size=1; yaw_rate output size=1; status input
function [phi,theta,psi,roll_rate,pitch_rate,yaw_rate] = fcn(data_uint8, status)
persistent stepp check_sum...
    phi_p theta_p psi_p roll_rate_p pitch_rate_p yaw_rate_p...
    phi_last theta_last psi_last roll_rate_last pitch_rate_last yaw_rate_last;
%% Initialize
if isempty(stepp)
    stepp=0;
    check_sum=0;
    phi_p=0;
    theta_p=0;
    psi_p=0;
    roll_rate_p=0;
    pitch_rate_p=0;
    yaw_rate_p=0;
    phi_last=0;
    theta_last=0;
    psi_last=0;
    roll_rate_last=0;
    pitch_rate_last=0;
    yaw_rate_last=0;
end
angle_scale=.0109863;  % 1/91.0222
rate_scale=1/16;
%% Check Each Byte
if status
    for i = 1:length(data_uint8)
        if (data_uint8(i)==115 && stepp==0)
            stepp=1;
            check_sum=data_uint8(i);
        elseif(stepp==1 && data_uint8(i)==110)
            stepp=stepp+1;
            check_sum=check_sum+data_uint8(i);
        elseif(stepp==2 && data_uint8(i)==112)
            stepp=stepp+1;
            check_sum=check_sum+data_uint8(i);
        elseif(stepp==3 && data_uint8(i)==212)
            stepp=stepp+1;
            check_sum=check_sum+data_uint8(i);
        elseif(stepp==4 && data_uint8(i)==112)
            stepp=stepp+1;
            check_sum=check_sum+data_uint8(i);
        elseif(stepp==5)
            phi_p=data_uint8(i)*256;
            stepp=stepp+1;
            check_sum=check_sum+data_uint8(i);
        elseif(stepp==6)
            phi_p=phi_p+data_uint8(i);
            stepp=stepp+1;
            check_sum=check_sum+data_uint8(i);
        elseif(stepp==7)
            theta_p=data_uint8(i)*256;
            stepp=stepp+1;
            check_sum=check_sum+data_uint8(i);
        elseif(stepp==8)
            theta_p=theta_p+data_uint8(i);
            stepp=stepp+1;
            check_sum=check_sum+data_uint8(i);
        elseif(stepp==9)
            psi_p=data_uint8(i)*256;
            stepp=stepp+1;
            check_sum=check_sum+data_uint8(i);
        elseif(stepp==10)
            psi_p=psi_p+data_uint8(i);
            stepp=stepp+1;
            check_sum=check_sum+data_uint8(i);
        elseif(stepp==11 || stepp==12)
            if(data_uint8(i)==0)
                stepp=stepp+1;
            else
                stepp=0;
            end
        elseif(stepp==13)
            roll_rate_p=data_uint8(i)*256;
            stepp=stepp+1;
            check_sum=check_sum+data_uint8(i);
        elseif(stepp==14)
            roll_rate_p=roll_rate_p+data_uint8(i);
            stepp=stepp+1;
            check_sum=check_sum+data_uint8(i);
        elseif(stepp==15)
            pitch_rate_p=data_uint8(i)*256;
            stepp=stepp+1;
            check_sum=check_sum+data_uint8(i);
        elseif(stepp==16)
            pitch_rate_p=pitch_rate_p+data_uint8(i);
            stepp=stepp+1;
            check_sum=check_sum+data_uint8(i);
        elseif(stepp==17)
            yaw_rate_p=data_uint8(i)*256;
            stepp=stepp+1;
            check_sum=check_sum+data_uint8(i);
        elseif(stepp==18)
            yaw_rate_p=yaw_rate_p+data_uint8(i);
            stepp=stepp+1;
            check_sum=check_sum+data_uint8(i);
        elseif(stepp==19 || stepp==20)
            if(data_uint8(i)==0)
                stepp=stepp+1;
            else
                stepp=0;
            end
        elseif(stepp==21 || stepp==22 || stepp==23 || stepp==24)
            stepp=stepp+1;
            check_sum=check_sum+data_uint8(i);
        elseif(stepp==25)
            if (floor(check_sum/256)==data_uint8(i))
                stepp=stepp+1;
            else
                stepp=0;
            end
        elseif(stepp==26)
            if(mod(check_sum,256)==data_uint8(i))
                phi_last=double(typecast(uint16(phi_p), 'int16'))*angle_scale;
                if mod(phi_last,360)>180
                    phi_last=mod(phi_last,360)-360;
                else
                    phi_last=mod(phi_last,360);
                end
                theta_last=double(typecast(uint16(theta_p), 'int16'))*angle_scale;
                if mod(theta_last,360)>180
                    theta_last=mod(theta_last,360)-360;
                else
                    theta_last=mod(theta_last,360);
                end
                psi_last=double(typecast(uint16(psi_p), 'int16'))*angle_scale;
                if mod(psi_last,360)>180
                    psi_last=mod(psi_last,360)-360;
                else
                    psi_last=mod(psi_last,360);
                end
                roll_rate_last=double(typecast(uint16(roll_rate_p), 'int16'))*rate_scale;
                if mod(roll_rate_last,360)>180
                    roll_rate_last=mod(roll_rate_last,360)-360;
                else
                    roll_rate_last=mod(roll_rate_last,360);
                end
                pitch_rate_last=double(typecast(uint16(pitch_rate_p), 'int16'))*rate_scale;
                if mod(pitch_rate_last,360)>180
                    pitch_rate_last=mod(pitch_rate_last,360)-360;
                else
                    pitch_rate_last=mod(pitch_rate_last,360);
                end
                yaw_rate_last=double(typecast(uint16(yaw_rate_p), 'int16'))*rate_scale;
                if mod(yaw_rate_last,360)>180
                    yaw_rate_last=mod(yaw_rate_last,360)-360;
                else
                    yaw_rate_last=mod(yaw_rate_last,360);
                end
            end
            stepp=0;
        end
    end
end

%% Assign Last True Data to Output
phi=phi_last-3;
theta=theta_last;
psi=psi_last;
roll_rate=roll_rate_last;
pitch_rate=pitch_rate_last;
yaw_rate=yaw_rate_last;

== matlab function PID_Yaw_2018b/Desired/MATLAB Function2 ==
  data: u input; y output
%% This Function Convert Inputs to [-180,180]
function y = fcn(u)
if mod(u,360)>180;
    y=mod(u,360)-360;
else
    y=mod(u,360);
end
end

== matlab function PID_Yaw_2018b/Desired/MATLAB Function1 ==
  data: u input; y output
%% This Function Convert Inputs to [-180,180]
function y = fcn(u)
if mod(u,360)>180;
    y=mod(u,360)-360;
else
    y=mod(u,360);
end
end

== matlab function PID_Yaw_2018b/Desired/MATLAB Function3 ==
  data: u input; y output
%% This Function Convert Inputs to [-180,180]
function y = fcn(u)
if mod(u,360)>180;
    y=mod(u,360)-360;
else
    y=mod(u,360);
end
end
